simulink model "example1"  (R2018b)
settings: Solver=FixedStepAuto  StartTime=0.0  StopTime=inf  RelTol=1e-3
libraries: aerolibanimutils x1
settings Model: Creator=Desktop-dds  LastModifiedBy=Desktop-dds

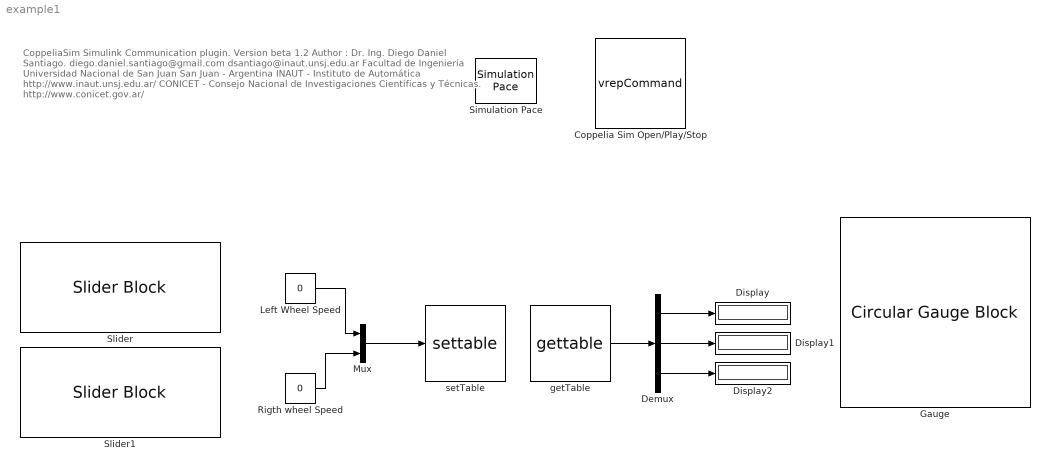
== system example1 ==
  note: CoppeliaSim Simulink Communication plugin.
      | Version beta 1.2
      | Author : Dr. Ing. Diego Daniel Santiago.
      | diego.daniel.santiago@gmail.com
      | dsantiago@inaut.unsj.edu.ar
      | Facultad de Ingeniería
      | Universidad Nacional de San Juan
      | San Juan - Argentina
      |
      | INAUT - Instituto de Automática
      | http://www.inaut.unsj.edu.ar/
      | CONICET - Consejo Nacional de Investigaciones Científicas y Técnicas.
      | http://www.conicet.gov.ar/
  Coppelia Sim Open/Play/Stop : S-Function  FunctionName=vrepCommand  Parameters=scene  SFunctionDeploymentMode=off  EnableBusSupport=off  mask{scene='example1.ttt'}
      mask prompts: scene "V-rep Scene Name"
      mask Display: image('play_stop.png')
  Demux : Demux  Outputs=3
  Display : Display
  Display1 : Display
  Display2 : Display
  Gauge : CircularGaugeBlock  WebBlockId=16  ScaleMax=1
  Left Wheel Speed : Constant  Value=0
  Mux : Mux  Inputs=2
  Rigth wheel Speed : Constant  Value=0
  Simulation Pace : aerolibanimutils/Simulation Pace  SimulationPace=1  SleepMode=Auto  OutputPaceError=off  SampleTime=1/30
  Slider : SliderBlock  WebBlockId=17  ScaleMax=5
  Slider1 : SliderBlock  WebBlockId=18  ScaleMax=5
  getTable : S-Function  FunctionName=gettable  Parameters=tname  SFunctionDeploymentMode=off  EnableBusSupport=off  mask{tname='sens'}
      mask prompts: tname "Table Name"
      mask DialogControl DescGroupVar Prompt: GetData
      mask DialogControl DescTextVar Prompt: Gets the data from a table declared in CoppeliaSim
      mask Display: image("CoppeliaSim.png")
  setTable : S-Function  FunctionName=settable  Parameters=tname  SFunctionDeploymentMode=off  EnableBusSupport=off  mask{tname='act'}
      mask prompts: tname "Table Name"
      mask DialogControl DescGroupVar Prompt: SetData
      mask DialogControl DescTextVar Prompt: Copy the input data into a table declared in CoppeliaSim
      mask Display: image("CoppeliaSim.png")
  wires:
  Mux/1 -> setTable/1
  Left Wheel Speed/1 -> Mux/1
  Rigth wheel Speed/1 -> Mux/2
  getTable/1 -> Demux/1
  Demux/1 -> Display/1
  Demux/2 -> Display1/1
  Demux/3 -> Display2/1
